simulink model "autopilot"  (R2020a)
settings: Solver=VariableStepAuto  StartTime=0.0  StopTime=400  RelTol=1e-3
values from neighbouring files (symbols this model uses):
  aileron_limit = deg2rad(30)    [Assignment2e.m]    (also in task1d.m)
  disturbance = deg2rad(1.5)    [Assignment2e.m]    (also in task1d.m)
  g = 9.81    [Assignment2e.m]    (also in task1d.m)
  kd_phi = (2*zeta_phi*omega_n_phi-a)/(b)    [Assignment2e.m]    (also in task1d.m)
  ki_phi = -0.15    [Assignment2e.m]    (also in task1d.m)
  ki_xi = omega_n_xi^2*Va/g    [Assignment2e.m]    (also in task1d.m)
  kp_phi = aileron_max/emax_phi*sign(b)    [Assignment2e.m]    (also in task1d.m)
  kp_xi = 2*zeta_xi*omega_n_xi*Va/g    [Assignment2e.m]    (also in task1d.m)
  Vg = Va    (= 580)    [Assignment2e.m]    (also in task1d.m)
undefined symbols (not defined in the file or in its folder): den, num
libraries: simulink x1
settings Model: Creator=henab  LastModifiedBy=henab

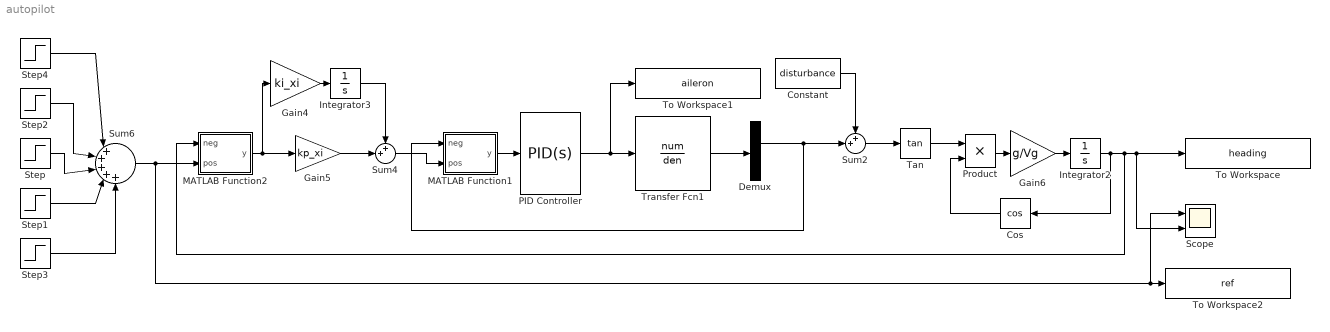
== system autopilot ==
  Constant : Constant  Value=disturbance
  Cos : Trigonometry  Operator=cos
  Demux : Demux
  Gain4 : Gain  Gain=ki_xi
  Gain5 : Gain  Gain=kp_xi
  Gain6 : Gain  Gain=g/Vg
  Integrator2 : Integrator
  Integrator3 : Integrator
  MATLAB Function1 : MATLAB Function  TreatAsAtomicUnit=on
  MATLAB Function2 : MATLAB Function  TreatAsAtomicUnit=on
  PID Controller : simulink/Continuous/PID Controller  Controller=PID  Form=Parallel  TimeDomain=Continuous-time  UseExternalTs=off  SampleTime=-1  IntegratorMethod=Forward Euler  FilterMethod=Forward Euler  ControllerParametersSource=internal  P=kp_phi  I=ki_phi  D=kd_phi  UseFilter=on  N=100  TunerSelectOption=Transfer Function Based (PID Tuner App)  InitialConditionSource=internal  InitialConditionForIntegrator=0  InitialConditionForFilter=0  DifferentiatorICPrevScaledInput=0  ExternalReset=none  TrackingMode=off  Kt=1  LimitOutput=on  UpperSaturationLimit=aileron_limit  LowerSaturationLimit=-aileron_limit  LinearizeAsGain=on  AntiWindupMode=back-calculation  Kb=1  POutMin=[]  POutMax=[]  IOutMin=[]  IOutMax=[]  DOutMin=[]  DOutMax=[]  NOutMin=[]  NOutMax=[]  SumOutMin=[]  SumOutMax=[]  SaturationOutMin=[]  SaturationOutMax=[]  PParamMin=[]  PParamMax=[]  IParamMin=[]  IParamMax=[]  DParamMin=[]  DParamMax=[]  NParamMin=[]  NParamMax=[]  KbParamMin=[]  KbParamMax=[]  KtParamMin=[]  KtParamMax=[]  KbOutMin=[]  KbOutMax=[]  KtOutMin=[]  KtOutMax=[]  IntegratorOutMin=[]  IntegratorOutMax=[]  FilterOutMin=[]  FilterOutMax=[]  SumI1OutMin=[]  SumI1OutMax=[]  SumI2OutMin=[]  SumI2OutMax=[]  SumI3OutMin=[]  SumI3OutMax=[]  SumI4OutMin=[]  SumI4OutMax=[]  SumDOutMin=[]  SumDOutMax=[]  DifferentiatorOutMin=[]  DifferentiatorOutMax=[]  FilterDiffOutCoefMin=[]  FilterDiffOutCoefMax=[]  ReciprocalOutMin=[]  ReciprocalOutMax=[]  SumDenOutMin=[]  SumDenOutMax=[]  SumNumOutMin=[]  SumNumOutMax=[]  DivideOutMin=[]  DivideOutMax=[]  UdiffTsProdOutMin=[]  UdiffTsProdOutMax=[]  NTsProdOutMin=[]  NTsProdOutMax=[]  UintegralTsProdOutMin=[]  UintegralTsProdOutMax=[]  UngainTsProdOutMin=[]  UngainTsProdOutMax=[]  IntegratorContinuousStateAttributes=''  IntegratorStateMustResolveToSignalObject=off  IntegratorRTWStateStorageClass=Auto  FilterContinuousStateAttributes=''  FilterStateMustResolveToSignalObject=off  FilterRTWStateStorageClass=Auto  ParallelPVariant=InternalParameters  IdealPVariant=Disabled  IVariant=InternalParameters  DVariant=InternalParameters  IntegratorVariant=Continuous  SatVariant=Enabled  AWVariant=BackCalculation  PCopyVariant=Disabled  TRVariant=Disabled  FdbkBlocksVariant=Forward  IdealPFdbkVariant=Disabled  SatFdbkVariant=Disabled  DerivativeFilterVariant=ContFilter  NVariant=InternalParameters  NCopyVariant=Disabled  FilterICVariant=InternalICsFilter  IntegratorICVariant=InternalICs  ExternalResetVariant=Disabled  TRSumVariant=Passthrough  SumFdbkVariant=Disabled  SumVariant=Sum_PID  TsampFilterVariant=InternalTs  TsampNgainVariant=Passthrough  TsampIntegralVariant=Passthrough
  Product : Product
  Scope : Scope  NumInputPorts=2
  Step : Step  Time=30  After=pi/12  SampleTime=0
  Step1 : Step  Time=50  After=-pi/24  SampleTime=0
  Step2 : Step  Time=150  After=-pi/6  SampleTime=0
  Step3 : Step  Time=180  After=pi/12  SampleTime=0
  Step4 : Step  Time=80  After=pi/12  SampleTime=0
  Sum2 : Sum  Inputs=++|
  Sum4 : Sum  Inputs=++|
  Sum6 : Sum  Inputs=|+++++
  Tan : Trigonometry  Operator=tan
  To Workspace : ToWorkspace  VariableName=heading  SaveFormat=Structure With Time  SampleTime=-1
  To Workspace1 : ToWorkspace  VariableName=aileron  SaveFormat=Structure With Time  SampleTime=-1
  To Workspace2 : ToWorkspace  VariableName=ref  SaveFormat=Structure With Time  SampleTime=-1
  Transfer Fcn1 : TransferFcn  Numerator=num  Denominator=den
  wires:
  Constant/1 -> Sum2/1
  Demux/2 -> MATLAB Function1/1(neg), Sum2/2
  MATLAB Function1/1(y) -> PID Controller/1
  Sum4/1 -> MATLAB Function1/2(pos)
  Gain4/1 -> Integrator3/1
  Integrator3/1 -> Sum4/1
  Gain5/1 -> Sum4/2
  MATLAB Function2/1(y) -> Gain4/1, Gain5/1
  PID Controller/1 -> To Workspace1/1, Transfer Fcn1/1
  Step4/1 -> Sum6/1
  Step2/1 -> Sum6/2
  Step/1 -> Sum6/3
  Step1/1 -> Sum6/4
  Step3/1 -> Sum6/5
  Sum6/1 -> MATLAB Function2/2(pos), Scope/1, To Workspace2/1
  Integrator2/1 -> Cos/1, MATLAB Function2/1(neg), To Workspace/1, Scope/2
  Transfer Fcn1/1 -> Demux/1
  Tan/1 -> Product/1
  Cos/1 -> Product/2
  Sum2/1 -> Tan/1
  Product/1 -> Gain6/1
  Gain6/1 -> Integrator2/1

== matlab function autopilot/MATLAB Function2 ==
  data: neg input; y output; pos input
function y = fcn(neg,pos)

y = angdiff(neg,pos);

== matlab function autopilot/MATLAB Function1 ==
  data: neg input; y output; pos input
function y = fcn(neg,pos)

y = angdiff(neg,pos);
